simulink model "NN_classification"  (R2015b)
settings: Solver=VariableStepAuto  StartTime=0.0  StopTime=10.0  RelTol=1e-3
values from neighbouring files (symbols this model uses):
  x3 = [VEa VEb VEc IEa IEb IEc V0 I0]    [final.m]    (also in final_online_classification.m = [va vb vc ia ib ic v0 i0]; final_online_detection.m = [va vb vc ia ib ic v0 i0]; final_online_detection1.m = [va vb vc ia ib ic v0 i0])
libraries: neural x108
(part 3 of 3)

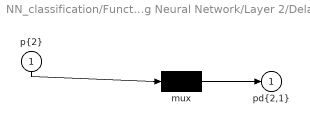
== system NN_classification/Function Fitting Neural Network/Layer 2/Delays 1 ==
  "p{2}" : Inport  PortDimensions=100
      mask Display: e = 0.06;c1 = [120 230 180]/255;c2 = ([120 230 180]+0)/(256+128);c3 = ([120 230 180]+128)/(256+128);patch([0 1 1 0],[0 0 1 1],c1);patch([0 1 1 1-e 1-e 0+e],[0 0 1 1-e 0+e 0+e],c2);patch([0 0 1 1-e 0+e 0+e],[0 1 1 1-e 1-e 0+e],c3);plot([0 1 1 0 0],[0 0 1 1 0]);
  mux : Mux  Inputs=1
      mask Display: e = 0.06;c1 = [120 150 230]/255;c2 = ([120 150 230]+0)/383;c3 = ([120 150 230]+128)/383;patch([0 1 1 0],[0 0 1 1],c1);patch([0 1 1 1-e 1-e 0+e],[0 0 1 1-e 0+e 0+e],c2);patch([0 0 1 1-e 0+e 0+e],[0 1 1 1-e 1-e 0+e],c3);plot([0 1 1 0 0],[0 0 1 1 0]);disp('Mux')
  "pd{2,1}" : Outport
      mask Display: e = 0.06;c1 = [120 230 180]/255;c2 = ([120 230 180]+0)/(256+128);c3 = ([120 230 180]+128)/(256+128);patch([0 1 1 0],[0 0 1 1],c1);patch([0 1 1 1-e 1-e 0+e],[0 0 1 1-e 0+e 0+e],c2);patch([0 0 1 1-e 0+e 0+e],[0 1 1 1-e 1-e 0+e],c3);plot([0 1 1 0 0],[0 0 1 1 0]);
  wires:
  "p{2}"/1 -> mux/1
  mux/1 -> "pd{2,1}"/1

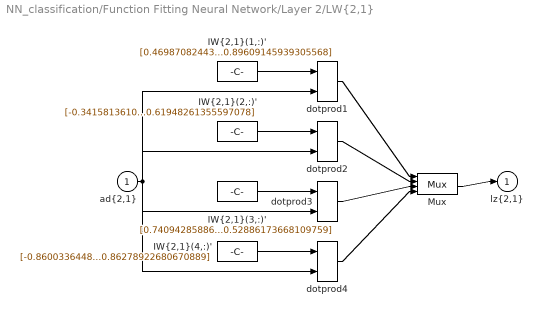
== system NN_classification/Function Fitting Neural Network/Layer 2/LW{2,1} ==
  "ad{2,1}" : Inport  PortDimensions=100
      mask Display: e = 0.06;c1 = [120 230 180]/255;c2 = ([120 230 180]+0)/(256+128);c3 = ([120 230 180]+128)/(256+128);patch([0 1 1 0],[0 0 1 1],c1);patch([0 1 1 1-e 1-e 0+e],[0 0 1 1-e 0+e 0+e],c2);patch([0 0 1 1-e 0+e 0+e],[0 1 1 1-e 1-e 0+e],c3);plot([0 1 1 0 0],[0 0 1 1 0]);
  "IW{2,1}(1,:)'" : Constant  Value=[0.46987082443325934;0.4885368747518905;0.18807319338392448;-0.62158299376365012;0.17677508244384632;-0.81625389346324773;-0.54074961000650867;-0.016489263238254163;0.76451985830305758;0.031337542569351361;0.32834435319978428;-0.72556398945990486;-0.6715467145184042;-0.12879190863899873;0.69358428259730853;-0.50747270890056873;0.44892948706838259;-0.54876965840504577;-0.84800171738465302;-0.045346124687123554;-0.44984558148540277;0.58299785545322236;0.75093849493652298;0.15601541954949896;-0.82806292817189986;-0.36628535626538195;0.89780717059509718;0.36769202525796002;0.061889426888160619;0.47977108846448402;-0.6786538026444825;-0.011599694663870045;-0.73031605639035746;0.76907135285336159;-0.30079734414532611;-0.3672967192257936;-0.077794830341673019;0.8453492969644214;-0.83186770970535617;0.26353739959433492;0.54153491667773423;-0.12335910717976412;-0.28701044638328255;0.92324393039828456;-0.11132733951959124;-0.87544209578356869;-0.61943776061707612;-1.038690040239582;-0.88719966194227307;0.58235508118562429;-0.15738279033798189;-0.38395136417430092;0.12115829107118499;0.69025133745460188;-0.20379309456103065;0.75083025643225521;0.099000779446309459;0.041744700708032725;-0.10155151990245248;0.55849426725114626;-0.85768359055614396;0.41229787862824174;-0.28823490976838911;-0.30908726931347313;-0.32228367347396741;-0.76510637014394656;0.4000131434867556;0.56739004313121155;-0.3358631484668137;-0.1477587433505394;-0.26532366135204832;-0.27889093464727166;0.050104144478982073;0.42168670486543702;-0.018939919762048358;0.65665102435761946;-0.027834183727619678;-0.19090649892610406;-0.86467544866727286;0.64452232334795234;0.47898212699879295;0.6343407427735368;0.54715180085504478;-0.79340770267522487;-0.83099068253515707;0.77664355301412569;-0.33855322720286724;-0.0454639132418692;-0.18003735792177969;-0.16386597470101449;0.16332540052320388;0.033267513100748561;-0.63862110630154312;0.46005369330709051;-0.58057221233403888;0.90957096002311788;-0.5232123095336173;0.54059696246036515;-0.7872678250824886;-0.89609145939305568]
      mask Display: e = 0.06;c1 = [120 150 230]/255;c2 = ([120 150 230]+0)/383;c3 = ([120 150 230]+128)/383;patch([0 1 1 0],[0 0 1 1],c1);patch([0 1 1 1-e 1-e 0+e],[0 0 1 1-e 0+e 0+e],c2);patch([0 0 1 1-e 0+e 0+e],[0 1 1 1-e 1-e 0+e],c3);plot([0 1 1 0 0],[0 0 1 1 0]);disp('weights');
  "IW{2,1}(2,:)'" : Constant  Value=[-0.34158136101295505;0.37055224423470751;-0.81954988188368127;-0.47347294209295088;0.14155902842373641;0.85335485060508742;0.19488003656446876;-0.75940568859668311;0.34874242563949542;0.96922629020562157;0.71359513183592693;0.61982446371929278;-0.1084466204878328;0.13602794275336372;0.0033199442952285101;0.26796342809942775;-0.37376269125240452;-0.47056995731449808;0.81144620318566318;0.37870484749264921;0.87292628479009682;-0.28882371655312317;-0.6435065151250563;0.2009286609218788;0.18228508337471946;0.88856941452179272;-0.65033231354368359;0.13395996770070842;-0.90800154762059215;-0.75470198171668412;0.72069755012993231;0.10156212899781497;-0.7889083595079277;-0.5719165794827572;0.50012496217317326;0.38340472833450234;0.76940952224723014;-0.36256953524828983;-0.4405240864412554;0.73439420694706137;-0.33427162136148492;0.58042009030306274;0.12064112131421756;-0.50274876932283019;-0.29692561184756278;-0.13213797788473958;0.18059409515873989;-0.68000169830062795;0.75218177866231073;0.79152503568458799;-0.4487683051902408;0.070430155645967912;-0.1915255726058572;-0.28870453685189745;0.44423860016563516;-0.49308763189143234;-0.78773420882500789;0.15132907505361443;-0.91189215443024019;-0.42576864208727838;0.84741296357541407;-0.1360886964489248;0.15700079942175432;0.58411875119656576;0.31646793020875624;0.046078175572039373;-0.2665163021947185;0.056943428558226539;-0.019883021023517029;-0.63719687563794125;-0.59250059630723129;-0.38025295051529839;0.65557435470092273;-0.72057072379583598;0.15878831524879441;0.57915649094521948;-0.46826384134391602;0.68525472075547189;-0.62964370378800794;0.027646775334377812;0.12904419136114206;-0.24069172667730435;0.65372694856586133;-0.87704515452116805;-0.25622945564155475;-0.35300240275771905;-0.58017871576045277;0.43363465073478219;0.80633456580847296;0.4522742096896849;0.43332234251085849;0.075392849220735692;-0.61745809185340172;0.52508522809898428;-0.15397075576300118;-0.090525924504402125;-0.15532979141662784;-0.18207153604807741;0.31406141476103472;0.61948261355597078]
      mask Display: e = 0.06;c1 = [120 150 230]/255;c2 = ([120 150 230]+0)/383;c3 = ([120 150 230]+128)/383;patch([0 1 1 0],[0 0 1 1],c1);patch([0 1 1 1-e 1-e 0+e],[0 0 1 1-e 0+e 0+e],c2);patch([0 0 1 1-e 0+e 0+e],[0 1 1 1-e 1-e 0+e],c3);plot([0 1 1 0 0],[0 0 1 1 0]);disp('weights');
  "IW{2,1}(3,:)'" : Constant  Value=[0.74094285886005495;-0.36977178928150251;0.38063703665447662;0.63646963663419509;0.24742774672071496;0.16631270368554518;0.49688985988779644;-0.71873649314266874;-0.019790195557011912;-0.59216829888989819;0.49167472387014349;0.57225177399313876;0.56957426870676409;-0.45370427794800461;-0.11930360732985654;0.59697506019170998;0.55738062405685951;-0.76131162653255768;0.50862443119232859;0.88026532857538675;-1.0016341641818072;-0.34698060199108233;-0.32693053158961971;0.2080819291759535;-0.86334739364054769;-0.45145084416143394;-0.68144164272690722;-0.83013964769454862;-0.76485354595302812;-0.59814735947100506;0.4111126917904363;-0.62333502325376511;-0.79732579167279161;-0.11094648760756558;0.2784976495897159;0.92038720671992591;-0.30988812477628563;-0.30369975787889547;0.29730263170474736;0.059117028101268322;0.36742198143746896;0.85175250924472434;0.94506990363287124;-0.66059574320586911;-0.33348594065787113;-0.37395666265284555;-0.274753332280606;-0.055525150156360274;-0.77306714875214577;-0.75638086990509701;0.047001934110895975;0.73304143831900959;-0.9436928240074266;-0.65058529742704907;-0.17541054581045576;-0.77811413923372708;0.75425262807209659;0.42539503244561006;0.78511952725694323;0.45152433944145759;-1.011193609080425;-0.30983798981055521;-0.74035707998357358;-0.40137522213435201;-0.70780816545595315;-0.86191768907349087;0.25528025617925826;0.57802187527356053;-0.70049924925175033;-0.051083868337177138;0.60952244595758021;-0.57839868313572929;-0.98613129882701811;0.73985256937228794;-0.9548633332556794;-0.034806119454187628;0.33466278787647641;0.52741886173729036;0.39778245700352244;-0.19134123617716581;0.020366485240295194;0.35500603491050781;0.85137230513597206;-0.76545119840950293;-0.22394642656734606;-0.23244699167624416;0.18624244715402063;0.25339205792848657;-0.73245024236672074;0.40300191667745255;-0.32201240979997114;0.11683756738150351;0.54433162889795794;0.62288202526858938;0.90761667517144828;-0.81092533962517999;0.31666062889144309;-0.45634715609515408;0.92816666629464439;-0.52886173668109759]
      mask Display: e = 0.06;c1 = [120 150 230]/255;c2 = ([120 150 230]+0)/383;c3 = ([120 150 230]+128)/383;patch([0 1 1 0],[0 0 1 1],c1);patch([0 1 1 1-e 1-e 0+e],[0 0 1 1-e 0+e 0+e],c2);patch([0 0 1 1-e 0+e 0+e],[0 1 1 1-e 1-e 0+e],c3);plot([0 1 1 0 0],[0 0 1 1 0]);disp('weights');
  "IW{2,1}(4,:)'" : Constant  Value=[-0.86003364481865041;3.2795463195073338;-1.5918244485562434;-1.8520959663501368;0.52859578962103437;0.39550003777832593;0.81909569794918813;1.0640757554356;1.4668340476536936;-2.6588731685019269;-0.32993221159858394;1.498161306123603;0.6653928667019301;0.92134375827311144;0.55128680003567576;0.72990923113533568;-1.597333761577818;0.25024559581720363;1.4958860080514598;0.83900754524121368;-0.7813670334548497;-0.4345676964133619;3.1570750221428288;-3.3169808395186138;0.11999855805420752;0.80271624156876831;-1.7430704330715903;1.5237566861436695;-1.6517327799865105;-0.58697968819671542;0.90283113885041744;-0.62522910447087199;1.5844123514611583;1.1204956873598986;-0.14269060182622312;1.1769696081695404;0.65134937508136803;1.8278404928912293;0.64091547993573372;1.1724127107448563;-0.71757505862925863;-0.02725647354899137;0.85502718154189905;-3.1305598982262111;0.23129669127873284;-0.30586139320746819;-0.55533885677681316;0.37659197708523379;0.5868244859963424;0.72745592654477376;2.4005499857346142;-1.0923891176064904;-0.71414248660365931;0.84188006894566703;0.084556844031949741;0.76848905927663147;-0.13996379150260091;0.42682412238132361;0.58662890812505197;-1.1926217001072643;2.1393443263547698;1.9138832222883104;-1.5060834468789053;-0.23998067167027254;0.62353698806336566;0.26827279159857037;2.3994753644366238;-0.79058785469503512;3.7384612624163625;-0.11488461012248632;0.60731616678449241;-3.4278847753481418;1.2453673555110336;-2.201574776663358;-1.9912496790262439;-1.1150448489501115;0.31119884753449684;2.4985775527275158;0.69103590793445524;1.4417000692928748;-1.1741813956930889;1.0709058411415371;1.4485832248631283;0.11086110863422022;-0.08074363609498085;4.3527431106041563;1.6862453492176941;-0.5543006765664259;-0.28465568635765637;0.44825003804058694;0.70723246329165834;-0.40951377233234171;-2.164648280126694;0.49140423050463689;0.46720894897813037;-0.47067051282872674;-0.24954761149245988;0.14545826179263452;-1.2053270491515207;-0.86278922680670889]
      mask Display: e = 0.06;c1 = [120 150 230]/255;c2 = ([120 150 230]+0)/383;c3 = ([120 150 230]+128)/383;patch([0 1 1 0],[0 0 1 1],c1);patch([0 1 1 1-e 1-e 0+e],[0 0 1 1-e 0+e 0+e],c2);patch([0 0 1 1-e 0+e 0+e],[0 1 1 1-e 1-e 0+e],c3);plot([0 1 1 0 0],[0 0 1 1 0]);disp('weights');
  Mux : Mux
      mask Display: e = 0.06;c1 = [120 150 230]/255;c2 = ([120 150 230]+0)/383;c3 = ([120 150 230]+128)/383;patch([0 1 1 0],[0 0 1 1],c1);patch([0 1 1 1-e 1-e 0+e],[0 0 1 1-e 0+e 0+e],c2);patch([0 0 1 1-e 0+e 0+e],[0 1 1 1-e 1-e 0+e],c3);plot([0 1 1 0 0],[0 0 1 1 0]);disp('Mux');
  dotprod{1..4} (4 alike) : neural/Weight Functions/dotprod
  "lz{2,1}" : Outport
      mask Display: e = 0.06;c1 = [120 230 180]/255;c2 = ([120 230 180]+0)/(256+128);c3 = ([120 230 180]+128)/(256+128);patch([0 1 1 0],[0 0 1 1],c1);patch([0 1 1 1-e 1-e 0+e],[0 0 1 1-e 0+e 0+e],c2);patch([0 0 1 1-e 0+e 0+e],[0 1 1 1-e 1-e 0+e],c3);plot([0 1 1 0 0],[0 0 1 1 0]);
  wires:
  "IW{2,1}(1,:)'"/1 -> dotprod1/1
  "ad{2,1}"/1 -> dotprod1/2, dotprod2/2, dotprod3/2, dotprod4/2
  dotprod1/1 -> Mux/1
  "IW{2,1}(2,:)'"/1 -> dotprod2/1
  dotprod2/1 -> Mux/2
  "IW{2,1}(3,:)'"/1 -> dotprod3/1
  dotprod3/1 -> Mux/3
  "IW{2,1}(4,:)'"/1 -> dotprod4/1
  dotprod4/1 -> Mux/4
  Mux/1 -> "lz{2,1}"/1
